simulink model "model"  (R2022a)
settings: Solver=VariableStepAuto  StartTime=0.0  StopTime=2  MaxStep=0.001  RelTol=1e-3
values from neighbouring files (symbols this model uses):
  A_d = sys_d.A    [tasks.m]
  B_d = sys_d.B    [tasks.m]
  K_d = K*inv(M)    [tasks.m]
  T = 0.2    [config.m]
  x_0 = [1; 0]    [tasks.m]
undefined symbols (not defined in the file or in its folder): A, B, C, L
settings Model: Creator=Vvlad  LastModifiedBy=Vvlad

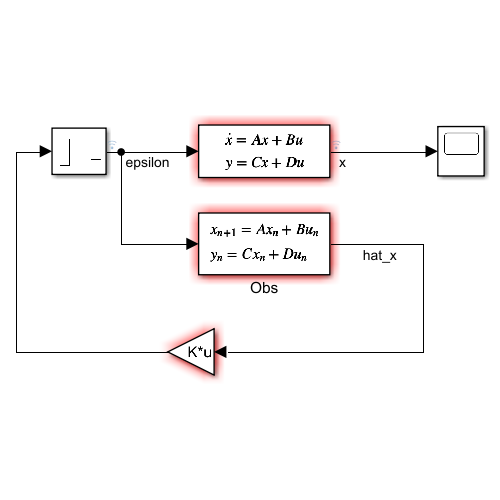
[thumbnail: Simulink's stored preview of the top-level diagram]
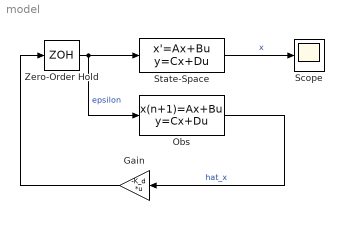
== system model ==
  Gain : Gain  Gain=-K_d  Multiplication=Matrix(K*u)
  Obs : DiscreteStateSpace  A=A_d - L*C  B=[B_d L]  C=eye(2)  D=0  SampleTime=T
  Scope : Scope
  State-Space : StateSpace  A=A  B=B  C=eye(2)  D=[0;0]  InitialCondition=x_0
  Zero-Order Hold : ZeroOrderHold  SampleTime=T
  wires:
  Gain/1 -> Zero-Order Hold/1
  State-Space/1 -> Scope/1  "x"
  Zero-Order Hold/1 -> Obs/1, State-Space/1  "epsilon"
  Obs/1 -> Gain/1  "hat_x"
